simulink model "WithLoad_Simple"  (R2017b)
settings: Solver=ode3  StartTime=0.0  StopTime=10  FixedStep=0.005  RelTol=1e-3  EnableMultiTasking=on
libraries: mblibv1 x61
(part 2 of 3)

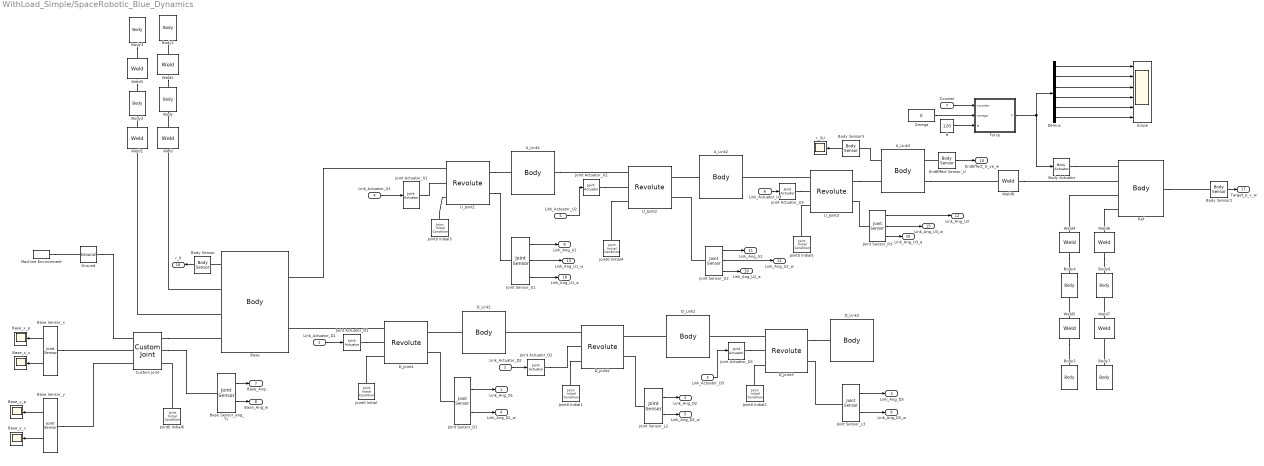
== system WithLoad_Simple/SpaceRobotic_Blue_Dynamics ==
  Link_Actuator_D1 : Inport
  Link_Actuator_D2 : Inport  Port=2
  Link_Actuator_D3 : Inport  Port=3
  Link_Actuator_U1 : Inport  Port=4
  Link_Actuator_U2 : Inport  Port=5
  Link_Actuator_U3 : Inport  Port=6
  Counter : Inport  Port=7
  Base : mblibv1/Bodies/Body  LConnTagsString=CG|CS14|CS15|CS1  RConnTagsString=CS16|CS17  UpdateFromCAD=off  DialogClass=MechanicalBodyBlock  Mass=44.0  MassUnits=kg  InertiaUnits=kg*m^2  Inertia=44.0*eye(3)  Shape=Cylinder  ShapeDims=[1 1]  ShapeUnits=m  ShapeUse=false  Density=1  DensityUnits=kg/m^3  DensityUse=false  GraphicsMode=MACHINE_DEFAULT  BodyColorSelMode=COLORPALETTE  BodyColor=[1 0.69412 0.39216]  AttachedToCS=CG  CG=Left$CG$[0.0 0 0]$CS1$CS1$m$[0 0 0]$Euler X-Y-Z$deg$WORLD$true$none  WorkingFrames=Left$CS14$[0 0 0.3]$CS1$CS1$m$[0 0 0]$Euler X-Y-Z$deg$WORLD$true$none#Left$CS15$[0 0 -0.3]$CS1$CS1$m$[0 0 0]$Euler X-Y-Z$deg$WORLD$true$none#Left$CS1$[0 0 0]$Adjoining$Adjoining$m$[0 0 0]$Euler X-Y-Z$deg$WORLD$true$none#Left$CS5$[-0.3 -0.3 0]$CS1$CS1$m$[0 0 0]$Euler X-Y-Z$deg$WORLD$false$none#Left$CS4$[-0.3 0.3 0]$CS1$CS1$m$[0 0 0]$Euler X-Y-Z$deg$WORLD$false$none#Right$CS2$[0.3 0.3 0]$CS1$CS1$m$[0 0 0]$Euler X-Y-Z$deg$WORLD$false$none#Right$CS16$[0.3 0.3 0]$CS1$CS1$m$[0 0 0]$Euler X-Y-Z$deg$WORLD$true$none#Right$CS3$[0.3 -0.3 0]$CS1$CS1$m$[0 0 0]$Euler X-Y-Z$deg$WORLD$false$none#Right$CS17$[0.3 -0.3 0]$CS1$CS1$m$[0 0 0]$Euler X-Y-Z$deg$WORLD$true$none#Right$CS13$[-0.3 0.3 -0.3]$CS1$CS1$m$[0 0 0]$Euler X-Y-Z$deg$WORLD$false$none#Right$CS12$[-0.3 0.3 0.3]$CS1$CS1$m$[0 0 0]$Euler X-Y-Z$deg$WORLD$false$none#Right$CS11$[0.3 0.3 -0.3]$CS1$CS1$m$[0 0 0]$Euler X-Y-Z$deg$WORLD$false$none#Right$CS10$[0.3 0.3 0.3]$CS1$CS1$m$[0 0 0]$Euler X-Y-Z$deg$WORLD$false$none#Right$CS9$[-0.3 -0.3 -0.3]$CS1$CS1$m$[0 0 0]$Euler X-Y-Z$deg$WORLD$false$none#Right$CS8$[0.3 -0.3 -0.3]$CS1$CS1$m$[0 0 0]$Euler X-Y-Z$deg$WORLD$false$none#Right$CS7$[-0.3 -0.3 0.3]$CS1$CS1$m$[0 0 0]$Euler X-Y-Z$deg$WORLD$false$none#Right$CS6$[0.3 -0.3 0.3]$CS1$CS1$m$[0 0 0]$Euler X-Y-Z$deg$WORLD$false$none  CGPos=[0.0 0 0]  CGRot=[0 0 0]  CS0Pos=[]  CS0Rot=[]  CS1Pos=[0 0 0]  CS1Rot=[0 0 0]  CS2Pos=[0.3 0.3 0]  CS2Rot=[0 0 0]  CS3Pos=[0.3 -0.3 0]  CS3Rot=[0 0 0]  CS4Pos=[-0.3 0.3 0]  CS4Rot=[0 0 0]  CS5Pos=[-0.3 -0.3 0]  CS5Rot=[0 0 0]  CS6Pos=[0.3 -0.3 0.3]  CS6Rot=[0 0 0]  CS7Pos=[-0.3 -0.3 0.3]  CS7Rot=[0 0 0]  CS8Pos=[0.3 -0.3 -0.3]  CS8Rot=[0 0 0]  CS9Pos=[-0.3 -0.3 -0.3]  CS9Rot=[0 0 0]  CS10Pos=[0.3 0.3 0.3]  CS10Rot=[0 0 0]  CS11Pos=[0.3 0.3 -0.3]  CS11Rot=[0 0 0]  CS12Pos=[-0.3 0.3 0.3]  CS12Rot=[0 0 0]  CS13Pos=[-0.3 0.3 -0.3]  CS13Rot=[0 0 0]  CS14Pos=[0 0 0.3]  CS14Rot=[0 0 0]  CS15Pos=[0 0 -0.3]  CS15Rot=[0 0 0]  CS16Pos=[0.3 0.3 0]  CS16Rot=[0 0 0]  CS17Pos=[0.3 -0.3 0]  CS17Rot=[0 0 0]  CS18Pos=[]  CS18Rot=[]  CS19Pos=[]  CS19Rot=[]  CS20Pos=[]  CS20Rot=[]
      settings: SourceProductName=Simscape Multibody  SourceProductBaseCode=MS
  Base Sensor_ang_Tc : mblibv1/Sensors &  Actuators/Joint Sensor  UpdateFromCAD=off  PhysicalDomain=Mechanical  PortType=blob  Muxed=off  Pose=off  Angle=on  AngleUnits=rad  ArcVelocity=on  ArcVelocityUnits=rad/s  ArcAcceleration=off  ArcAccelerationUnits=deg/s^2  CoordPosition=on  CoordPositionUnits=m  Velocity=off  VelocityUnits=m/s  Acceleration=off  AccelerationUnits=m/s^2  Quaternion=on  QuaternionDT=off  QuaternionDDT=off  QuaternionUnits=off  OutputVector=[1]  ActiveIO=on  Width=2  DialogClass=MechanicalSensorBlock  Primitive=R1  Force=off  ForceUnits=N  Torque=off  TorqueUnits=N*m  ReferenceFrame=Absolute (World)  ReactionSensedSide=Base  ReactionReferenceFrame=Absolute (World)  ReactionForce=off  ReactionForceUnits=N  ReactionMoment=off  ReactionMomentUnits=N*m
      settings: SourceProductName=Simscape Multibody  SourceProductBaseCode=MS
  Base Sensor_x : mblibv1/Sensors &  Actuators/Joint Sensor  UpdateFromCAD=off  PhysicalDomain=Mechanical  PortType=blob  Muxed=off  Pose=off  Angle=on  AngleUnits=deg  ArcVelocity=on  ArcVelocityUnits=deg/s  ArcAcceleration=off  ArcAccelerationUnits=deg/s^2  CoordPosition=on  CoordPositionUnits=m  Velocity=on  VelocityUnits=m/s  Acceleration=off  AccelerationUnits=m/s^2  Quaternion=on  QuaternionDT=off  QuaternionDDT=off  QuaternionUnits=off  OutputVector=[1]  ActiveIO=on  Width=2  DialogClass=MechanicalSensorBlock  Primitive=P1  Force=off  ForceUnits=N  Torque=off  TorqueUnits=N*m  ReferenceFrame=Absolute (World)  ReactionSensedSide=Base  ReactionReferenceFrame=Absolute (World)  ReactionForce=off  ReactionForceUnits=N  ReactionMoment=off  ReactionMomentUnits=N*m
      settings: SourceProductName=Simscape Multibody  SourceProductBaseCode=MS
  Base Sensor_y : mblibv1/Sensors &  Actuators/Joint Sensor  UpdateFromCAD=off  PhysicalDomain=Mechanical  PortType=blob  Muxed=off  Pose=off  Angle=on  AngleUnits=deg  ArcVelocity=on  ArcVelocityUnits=deg/s  ArcAcceleration=off  ArcAccelerationUnits=deg/s^2  CoordPosition=on  CoordPositionUnits=m  Velocity=on  VelocityUnits=m/s  Acceleration=off  AccelerationUnits=m/s^2  Quaternion=on  QuaternionDT=off  QuaternionDDT=off  QuaternionUnits=off  OutputVector=[1]  ActiveIO=on  Width=2  DialogClass=MechanicalSensorBlock  Primitive=P2  Force=off  ForceUnits=N  Torque=off  TorqueUnits=N*m  ReferenceFrame=Absolute (World)  ReactionSensedSide=Base  ReactionReferenceFrame=Absolute (World)  ReactionForce=off  ReactionForceUnits=N  ReactionMoment=off  ReactionMomentUnits=N*m
      settings: SourceProductName=Simscape Multibody  SourceProductBaseCode=MS
  Base_x_p : Scope
  Base_x_v : Scope
  Base_y_p : Scope
  Base_y_v : Scope
  Body : mblibv1/Bodies/Body  LConnTagsString=CS1  RConnTagsString=CS2  UpdateFromCAD=off  DialogClass=MechanicalBodyBlock  Mass=1*0.00001  MassUnits=kg  InertiaUnits=kg*m^2  Inertia=eye(3)*0.00001*(1)  Shape=Cylinder  ShapeDims=[1 1]  ShapeUnits=m  ShapeUse=false  Density=1  DensityUnits=kg/m^3  DensityUse=false  GraphicsMode=MACHINE_DEFAULT  BodyColorSelMode=COLORPALETTE  BodyColor=[0 0 1]  AttachedToCS=CG  CG=Left$CG$[0 0 0.1]$CS1$CS1$m$[0 0 0]$Euler X-Y-Z$deg$WORLD$false$none  WorkingFrames=Left$CS1$[0 0 0]$Adjoining$Adjoining$m$[0 0 0]$Euler X-Y-Z$deg$WORLD$true$none#Right$CS2$[0 0 0.2]$CS1$CS1$m$[0 0 0]$Euler X-Y-Z$deg$WORLD$true$none  CGPos=[0 0 0.1]  CGRot=[0 0 0]  CS0Pos=[]  CS0Rot=[]  CS1Pos=[0 0 0]  CS1Rot=[0 0 0]  CS2Pos=[0 0 0.2]  CS2Rot=[0 0 0]  CS3Pos=[]  CS3Rot=[]  CS4Pos=[]  CS4Rot=[]  CS5Pos=[]  CS5Rot=[]  CS6Pos=[]  CS6Rot=[]  CS7Pos=[]  CS7Rot=[]  CS8Pos=[]  CS8Rot=[]  CS9Pos=[]  CS9Rot=[]  CS10Pos=[]  CS10Rot=[]  CS11Pos=[]  CS11Rot=[]  CS12Pos=[]  CS12Rot=[]  CS13Pos=[]  CS13Rot=[]  CS14Pos=[]  CS14Rot=[]  CS15Pos=[]  CS15Rot=[]  CS16Pos=[]  CS16Rot=[]  CS17Pos=[]  CS17Rot=[]  CS18Pos=[]  CS18Rot=[]  CS19Pos=[]  CS19Rot=[]  CS20Pos=[]  CS20Rot=[]
      settings: SourceProductName=Simscape Multibody  SourceProductBaseCode=MS
  Body Actuator : mblibv1/Sensors &  Actuators/Body Actuator  UpdateFromCAD=off  PhysicalDomain=Mechanical  PortType=blob  ActuationStyle=Force  AngleUnits=deg  ArcVelocityUnits=deg/s  ArcAccelerationUnits=deg/s^2  CoordPositionUnits=m  VelocityUnits=m/s  AccelerationUnits=m/s^2  ForceUnits=N  TorqueUnits=N*m  ActiveIO=on  Width=6  DialogClass=MechanicalActuatorBlock  ReferenceFrame=Local (Body CS)  Angle=off  CoordPosition=on  Force=on  Torque=on
      settings: SourceProductName=Simscape Multibody  SourceProductBaseCode=MS
  Body Sensor : mblibv1/Sensors &  Actuators/Body Sensor  UpdateFromCAD=off  PhysicalDomain=Mechanical  PortType=blob  Muxed=on  Pose=off  Angle=on  AngleUnits=deg  ArcVelocity=on  ArcVelocityUnits=rad/s  ArcAcceleration=on  ArcAccelerationUnits=deg/s^2  CoordPosition=on  CoordPositionUnits=m  Velocity=on  VelocityUnits=m/s  Acceleration=off  AccelerationUnits=m/s^2  Quaternion=on  QuaternionDT=off  QuaternionDDT=off  QuaternionUnits=off  OutputVector=[1]  ActiveIO=on  Width=12  DialogClass=MechanicalSensorBlock  ReferenceFrame=Absolute (World)
      settings: SourceProductName=Simscape Multibody  SourceProductBaseCode=MS
  Body Sensor2 : mblibv1/Sensors &  Actuators/Body Sensor  UpdateFromCAD=off  PhysicalDomain=Mechanical  PortType=blob  Muxed=on  Pose=off  Angle=on  AngleUnits=deg  ArcVelocity=on  ArcVelocityUnits=rad/s  ArcAcceleration=off  ArcAccelerationUnits=deg/s^2  CoordPosition=on  CoordPositionUnits=m  Velocity=on  VelocityUnits=m/s  Acceleration=off  AccelerationUnits=m/s^2  Quaternion=on  QuaternionDT=off  QuaternionDDT=off  QuaternionUnits=off  OutputVector=[1]  ActiveIO=on  Width=9  DialogClass=MechanicalSensorBlock  ReferenceFrame=Absolute (World)
      settings: SourceProductName=Simscape Multibody  SourceProductBaseCode=MS
  Body Sensor5 : mblibv1/Sensors &  Actuators/Body Sensor  UpdateFromCAD=off  PhysicalDomain=Mechanical  PortType=blob  Muxed=on  Pose=off  Angle=on  AngleUnits=deg  ArcVelocity=off  ArcVelocityUnits=deg/s  ArcAcceleration=off  ArcAccelerationUnits=deg/s^2  CoordPosition=on  CoordPositionUnits=m  Velocity=off  VelocityUnits=m/s  Acceleration=off  AccelerationUnits=m/s^2  Quaternion=on  QuaternionDT=off  QuaternionDDT=off  QuaternionUnits=off  OutputVector=[1]  ActiveIO=on  Width=3  DialogClass=MechanicalSensorBlock  ReferenceFrame=Absolute (World)
      settings: SourceProductName=Simscape Multibody  SourceProductBaseCode=MS
  Body1 : mblibv1/Bodies/Body  LConnTagsString=CS1  UpdateFromCAD=off  DialogClass=MechanicalBodyBlock  Mass=1*0.00001  MassUnits=kg  InertiaUnits=kg*m^2  Inertia=eye(3)*0.00001  Shape=Cylinder  ShapeDims=[1 1]  ShapeUnits=m  ShapeUse=false  Density=1  DensityUnits=kg/m^3  DensityUse=false  GraphicsMode=MACHINE_DEFAULT  BodyColorSelMode=COLORPALETTE  BodyColor=[0 0 1]  AttachedToCS=CG  CG=Left$CG$[0 0 0.45]$CS1$CS1$m$[0 0 0]$Euler X-Y-Z$deg$WORLD$false$none  WorkingFrames=Left$CS1$[0 0 0]$Adjoining$Adjoining$m$[0 0 0]$Euler X-Y-Z$deg$WORLD$true$none#Right$CS2$[0.2 0.01 0]$CS1$CS1$m$[0 0 0]$Euler X-Y-Z$deg$WORLD$false$none#Right$CS3$[0.2 -0.01 0]$CS1$CS1$m$[0 0 0]$Euler X-Y-Z$deg$WORLD$false$none#Right$CS4$[-0.2 0.01 0]$CS1$CS1$m$[0 0 0]$Euler X-Y-Z$deg$WORLD$false$none#Right$CS5$[-0.2 -0.01 0]$CS1$CS1$m$[0 0 0]$Euler X-Y-Z$deg$WORLD$false$none#Right$CS6$[-0.2 -0.01 0.9]$CS1$CS1$m$[0 0 0]$Euler X-Y-Z$deg$WORLD$false$none#Right$CS7$[-0.2 0.01 0.9]$CS1$CS1$m$[0 0 0]$Euler X-Y-Z$deg$WORLD$false$none#Right$CS8$[0.2 0.01 0.9]$CS1$CS1$m$[0 0 0]$Euler X-Y-Z$deg$WORLD$false$none#Right$CS9$[0.2 -0.01 0.9]$CS1$CS1$m$[0 0 0]$Euler X-Y-Z$deg$WORLD$false$none  CGPos=[0 0 0.45]  CGRot=[0 0 0]  CS0Pos=[]  CS0Rot=[]  CS1Pos=[0 0 0]  CS1Rot=[0 0 0]  CS2Pos=[0.2 0.01 0]  CS2Rot=[0 0 0]  CS3Pos=[0.2 -0.01 0]  CS3Rot=[0 0 0]  CS4Pos=[-0.2 0.01 0]  CS4Rot=[0 0 0]  CS5Pos=[-0.2 -0.01 0]  CS5Rot=[0 0 0]  CS6Pos=[-0.2 -0.01 0.9]  CS6Rot=[0 0 0]  CS7Pos=[-0.2 0.01 0.9]  CS7Rot=[0 0 0]  CS8Pos=[0.2 0.01 0.9]  CS8Rot=[0 0 0]  CS9Pos=[0.2 -0.01 0.9]  CS9Rot=[0 0 0]  CS10Pos=[]  CS10Rot=[]  CS11Pos=[]  CS11Rot=[]  CS12Pos=[]  CS12Rot=[]  CS13Pos=[]  CS13Rot=[]  CS14Pos=[]  CS14Rot=[]  CS15Pos=[]  CS15Rot=[]  CS16Pos=[]  CS16Rot=[]  CS17Pos=[]  CS17Rot=[]  CS18Pos=[]  CS18Rot=[]  CS19Pos=[]  CS19Rot=[]  CS20Pos=[]  CS20Rot=[]
      settings: SourceProductName=Simscape Multibody  SourceProductBaseCode=MS
  Body2 : mblibv1/Bodies/Body  LConnTagsString=CS1  RConnTagsString=CS2  UpdateFromCAD=off  DialogClass=MechanicalBodyBlock  Mass=1*0.00001  MassUnits=kg  InertiaUnits=kg*m^2  Inertia=eye(3)*0.00001  Shape=Cylinder  ShapeDims=[1 1]  ShapeUnits=m  ShapeUse=false  Density=1  DensityUnits=kg/m^3  DensityUse=false  GraphicsMode=MACHINE_DEFAULT  BodyColorSelMode=COLORPALETTE  BodyColor=[0 0 1]  AttachedToCS=CG  CG=Left$CG$[0 0 -0.1]$CS1$CS1$m$[0 0 0]$Euler X-Y-Z$deg$WORLD$false$none  WorkingFrames=Left$CS1$[0 0 0]$Adjoining$Adjoining$m$[0 0 0]$Euler X-Y-Z$deg$WORLD$true$none#Right$CS2$[0 0 -0.2]$CS1$CS1$m$[0 0 0]$Euler X-Y-Z$deg$WORLD$true$none  CGPos=[0 0 -0.1]  CGRot=[0 0 0]  CS0Pos=[]  CS0Rot=[]  CS1Pos=[0 0 0]  CS1Rot=[0 0 0]  CS2Pos=[0 0 -0.2]  CS2Rot=[0 0 0]  CS3Pos=[]  CS3Rot=[]  CS4Pos=[]  CS4Rot=[]  CS5Pos=[]  CS5Rot=[]  CS6Pos=[]  CS6Rot=[]  CS7Pos=[]  CS7Rot=[]  CS8Pos=[]  CS8Rot=[]  CS9Pos=[]  CS9Rot=[]  CS10Pos=[]  CS10Rot=[]  CS11Pos=[]  CS11Rot=[]  CS12Pos=[]  CS12Rot=[]  CS13Pos=[]  CS13Rot=[]  CS14Pos=[]  CS14Rot=[]  CS15Pos=[]  CS15Rot=[]  CS16Pos=[]  CS16Rot=[]  CS17Pos=[]  CS17Rot=[]  CS18Pos=[]  CS18Rot=[]  CS19Pos=[]  CS19Rot=[]  CS20Pos=[]  CS20Rot=[]
      settings: SourceProductName=Simscape Multibody  SourceProductBaseCode=MS
  Body3 : mblibv1/Bodies/Body  LConnTagsString=CS1  UpdateFromCAD=off  DialogClass=MechanicalBodyBlock  Mass=1*0.00001  MassUnits=kg  InertiaUnits=kg*m^2  Inertia=eye(3)*0.00001  Shape=Cylinder  ShapeDims=[1 1]  ShapeUnits=m  ShapeUse=false  Density=1  DensityUnits=kg/m^3  DensityUse=false  GraphicsMode=MACHINE_DEFAULT  BodyColorSelMode=COLORPALETTE  BodyColor=[0 0 1]  AttachedToCS=CG  CG=Left$CG$[0 0 0.45]$CS1$CS1$m$[0 0 0]$Euler X-Y-Z$deg$WORLD$false$none  WorkingFrames=Left$CS1$[0 0 0]$Adjoining$Adjoining$m$[0 0 0]$Euler X-Y-Z$deg$WORLD$true$none#Right$CS2$[0.2 0.01 0]$CS1$CS1$m$[0 0 0]$Euler X-Y-Z$deg$WORLD$false$none#Right$CS3$[0.2 -0.01 0]$CS1$CS1$m$[0 0 0]$Euler X-Y-Z$deg$WORLD$false$none#Right$CS4$[-0.2 0.01 0]$CS1$CS1$m$[0 0 0]$Euler X-Y-Z$deg$WORLD$false$none#Right$CS5$[-0.2 -0.01 0]$CS1$CS1$m$[0 0 0]$Euler X-Y-Z$deg$WORLD$false$none#Right$CS6$[-0.2 -0.01 -0.9]$CS1$CS1$m$[0 0 0]$Euler X-Y-Z$deg$WORLD$false$none#Right$CS7$[-0.2 0.01 -0.9]$CS1$CS1$m$[0 0 0]$Euler X-Y-Z$deg$WORLD$false$none#Right$CS8$[0.2 0.01 -0.9]$CS1$CS1$m$[0 0 0]$Euler X-Y-Z$deg$WORLD$false$none#Right$CS9$[0.2 -0.01 -0.9]$CS1$CS1$m$[0 0 0]$Euler X-Y-Z$deg$WORLD$false$none  CGPos=[0 0 0.45]  CGRot=[0 0 0]  CS0Pos=[]  CS0Rot=[]  CS1Pos=[0 0 0]  CS1Rot=[0 0 0]  CS2Pos=[0.2 0.01 0]  CS2Rot=[0 0 0]  CS3Pos=[0.2 -0.01 0]  CS3Rot=[0 0 0]  CS4Pos=[-0.2 0.01 0]  CS4Rot=[0 0 0]  CS5Pos=[-0.2 -0.01 0]  CS5Rot=[0 0 0]  CS6Pos=[-0.2 -0.01 -0.9]  CS6Rot=[0 0 0]  CS7Pos=[-0.2 0.01 -0.9]  CS7Rot=[0 0 0]  CS8Pos=[0.2 0.01 -0.9]  CS8Rot=[0 0 0]  CS9Pos=[0.2 -0.01 -0.9]  CS9Rot=[0 0 0]  CS10Pos=[]  CS10Rot=[]  CS11Pos=[]  CS11Rot=[]  CS12Pos=[]  CS12Rot=[]  CS13Pos=[]  CS13Rot=[]  CS14Pos=[]  CS14Rot=[]  CS15Pos=[]  CS15Rot=[]  CS16Pos=[]  CS16Rot=[]  CS17Pos=[]  CS17Rot=[]  CS18Pos=[]  CS18Rot=[]  CS19Pos=[]  CS19Rot=[]  CS20Pos=[]  CS20Rot=[]
      settings: SourceProductName=Simscape Multibody  SourceProductBaseCode=MS
  Body4 : mblibv1/Bodies/Body  LConnTagsString=CS1  RConnTagsString=CS2  UpdateFromCAD=off  DialogClass=MechanicalBodyBlock  Mass=1*0.00001  MassUnits=kg  InertiaUnits=kg*m^2  Inertia=eye(3)*0.00001  Shape=Cylinder  ShapeDims=[1 1]  ShapeUnits=m  ShapeUse=false  Density=1  DensityUnits=kg/m^3  DensityUse=false  GraphicsMode=MACHINE_DEFAULT  BodyColorSelMode=COLORPALETTE  BodyColor=[0 0 1]  AttachedToCS=CG  CG=Left$CG$[0 0 0.1]$CS1$CS1$m$[0 0 0]$Euler X-Y-Z$deg$WORLD$false$none  WorkingFrames=Left$CS1$[0 0 0]$Adjoining$Adjoining$m$[0 0 0]$Euler X-Y-Z$deg$WORLD$true$none#Right$CS2$[0 0 0.2]$CS1$CS1$m$[0 0 0]$Euler X-Y-Z$deg$WORLD$true$none  CGPos=[0 0 0.1]  CGRot=[0 0 0]  CS0Pos=[]  CS0Rot=[]  CS1Pos=[0 0 0]  CS1Rot=[0 0 0]  CS2Pos=[0 0 0.2]  CS2Rot=[0 0 0]  CS3Pos=[]  CS3Rot=[]  CS4Pos=[]  CS4Rot=[]  CS5Pos=[]  CS5Rot=[]  CS6Pos=[]  CS6Rot=[]  CS7Pos=[]  CS7Rot=[]  CS8Pos=[]  CS8Rot=[]  CS9Pos=[]  CS9Rot=[]  CS10Pos=[]  CS10Rot=[]  CS11Pos=[]  CS11Rot=[]  CS12Pos=[]  CS12Rot=[]  CS13Pos=[]  CS13Rot=[]  CS14Pos=[]  CS14Rot=[]  CS15Pos=[]  CS15Rot=[]  CS16Pos=[]  CS16Rot=[]  CS17Pos=[]  CS17Rot=[]  CS18Pos=[]  CS18Rot=[]  CS19Pos=[]  CS19Rot=[]  CS20Pos=[]  CS20Rot=[]
      settings: SourceProductName=Simscape Multibody  SourceProductBaseCode=MS
  Body5 : mblibv1/Bodies/Body  LConnTagsString=CS1  UpdateFromCAD=off  DialogClass=MechanicalBodyBlock  Mass=1*0.00001  MassUnits=kg  InertiaUnits=kg*m^2  Inertia=eye(3)*0.00001  Shape=Cylinder  ShapeDims=[1 1]  ShapeUnits=m  ShapeUse=false  Density=1  DensityUnits=kg/m^3  DensityUse=false  GraphicsMode=MACHINE_DEFAULT  BodyColorSelMode=COLORPALETTE  BodyColor=[0 0 1]  AttachedToCS=CG  CG=Left$CG$[0 0 0.45]$CS1$CS1$m$[0 0 0]$Euler X-Y-Z$deg$WORLD$false$none  WorkingFrames=Left$CS1$[0 0 0]$Adjoining$Adjoining$m$[0 0 0]$Euler X-Y-Z$deg$WORLD$true$none#Right$CS2$[0.2 0.01 0]$CS1$CS1$m$[0 0 0]$Euler X-Y-Z$deg$WORLD$false$none#Right$CS3$[0.2 -0.01 0]$CS1$CS1$m$[0 0 0]$Euler X-Y-Z$deg$WORLD$false$none#Right$CS4$[-0.2 0.01 0]$CS1$CS1$m$[0 0 0]$Euler X-Y-Z$deg$WORLD$false$none#Right$CS5$[-0.2 -0.01 0]$CS1$CS1$m$[0 0 0]$Euler X-Y-Z$deg$WORLD$false$none#Right$CS6$[-0.2 -0.01 1]$CS1$CS1$m$[0 0 0]$Euler X-Y-Z$deg$WORLD$false$none#Right$CS7$[-0.2 0.01 1]$CS1$CS1$m$[0 0 0]$Euler X-Y-Z$deg$WORLD$false$none#Right$CS8$[0.2 0.01 1]$CS1$CS1$m$[0 0 0]$Euler X-Y-Z$deg$WORLD$false$none#Right$CS9$[0.2 -0.01 1]$CS1$CS1$m$[0 0 0]$Euler X-Y-Z$deg$WORLD$false$none  CGPos=[0 0 0.45]  CGRot=[0 0 0]  CS0Pos=[]  CS0Rot=[]  CS1Pos=[0 0 0]  CS1Rot=[0 0 0]  CS2Pos=[0.2 0.01 0]  CS2Rot=[0 0 0]  CS3Pos=[0.2 -0.01 0]  CS3Rot=[0 0 0]  CS4Pos=[-0.2 0.01 0]  CS4Rot=[0 0 0]  CS5Pos=[-0.2 -0.01 0]  CS5Rot=[0 0 0]  CS6Pos=[-0.2 -0.01 1]  CS6Rot=[0 0 0]  CS7Pos=[-0.2 0.01 1]  CS7Rot=[0 0 0]  CS8Pos=[0.2 0.01 1]  CS8Rot=[0 0 0]  CS9Pos=[0.2 -0.01 1]  CS9Rot=[0 0 0]  CS10Pos=[]  CS10Rot=[]  CS11Pos=[]  CS11Rot=[]  CS12Pos=[]  CS12Rot=[]  CS13Pos=[]  CS13Rot=[]  CS14Pos=[]  CS14Rot=[]  CS15Pos=[]  CS15Rot=[]  CS16Pos=[]  CS16Rot=[]  CS17Pos=[]  CS17Rot=[]  CS18Pos=[]  CS18Rot=[]  CS19Pos=[]  CS19Rot=[]  CS20Pos=[]  CS20Rot=[]
      settings: SourceProductName=Simscape Multibody  SourceProductBaseCode=MS
  Body6 : mblibv1/Bodies/Body  LConnTagsString=CS1  RConnTagsString=CS2  UpdateFromCAD=off  DialogClass=MechanicalBodyBlock  Mass=1*0.00001  MassUnits=kg  InertiaUnits=kg*m^2  Inertia=eye(3)*0.00001  Shape=Cylinder  ShapeDims=[1 1]  ShapeUnits=m  ShapeUse=false  Density=1  DensityUnits=kg/m^3  DensityUse=false  GraphicsMode=MACHINE_DEFAULT  BodyColorSelMode=COLORPALETTE  BodyColor=[0 0 1]  AttachedToCS=CG  CG=Left$CG$[0 0 -0.1]$CS1$CS1$m$[0 0 0]$Euler X-Y-Z$deg$WORLD$false$none  WorkingFrames=Left$CS1$[0 0 0]$Adjoining$Adjoining$m$[0 0 0]$Euler X-Y-Z$deg$WORLD$true$none#Right$CS2$[0 0 -0.2]$CS1$CS1$m$[0 0 0]$Euler X-Y-Z$deg$WORLD$true$none  CGPos=[0 0 -0.1]  CGRot=[0 0 0]  CS0Pos=[]  CS0Rot=[]  CS1Pos=[0 0 0]  CS1Rot=[0 0 0]  CS2Pos=[0 0 -0.2]  CS2Rot=[0 0 0]  CS3Pos=[]  CS3Rot=[]  CS4Pos=[]  CS4Rot=[]  CS5Pos=[]  CS5Rot=[]  CS6Pos=[]  CS6Rot=[]  CS7Pos=[]  CS7Rot=[]  CS8Pos=[]  CS8Rot=[]  CS9Pos=[]  CS9Rot=[]  CS10Pos=[]  CS10Rot=[]  CS11Pos=[]  CS11Rot=[]  CS12Pos=[]  CS12Rot=[]  CS13Pos=[]  CS13Rot=[]  CS14Pos=[]  CS14Rot=[]  CS15Pos=[]  CS15Rot=[]  CS16Pos=[]  CS16Rot=[]  CS17Pos=[]  CS17Rot=[]  CS18Pos=[]  CS18Rot=[]  CS19Pos=[]  CS19Rot=[]  CS20Pos=[]  CS20Rot=[]
      settings: SourceProductName=Simscape Multibody  SourceProductBaseCode=MS
  Body7 : mblibv1/Bodies/Body  LConnTagsString=CS1  UpdateFromCAD=off  DialogClass=MechanicalBodyBlock  Mass=1*0.00001  MassUnits=kg  InertiaUnits=kg*m^2  Inertia=eye(3)*0.00001  Shape=Cylinder  ShapeDims=[1 1]  ShapeUnits=m  ShapeUse=false  Density=1  DensityUnits=kg/m^3  DensityUse=false  GraphicsMode=MACHINE_DEFAULT  BodyColorSelMode=COLORPALETTE  BodyColor=[0 0 1]  AttachedToCS=CG  CG=Left$CG$[0 0 0.45]$CS1$CS1$m$[0 0 0]$Euler X-Y-Z$deg$WORLD$false$none  WorkingFrames=Left$CS1$[0 0 0]$Adjoining$Adjoining$m$[0 0 0]$Euler X-Y-Z$deg$WORLD$true$none#Right$CS2$[0.2 0.01 0]$CS1$CS1$m$[0 0 0]$Euler X-Y-Z$deg$WORLD$false$none#Right$CS3$[0.2 -0.01 0]$CS1$CS1$m$[0 0 0]$Euler X-Y-Z$deg$WORLD$false$none#Right$CS4$[-0.2 0.01 0]$CS1$CS1$m$[0 0 0]$Euler X-Y-Z$deg$WORLD$false$none#Right$CS5$[-0.2 -0.01 0]$CS1$CS1$m$[0 0 0]$Euler X-Y-Z$deg$WORLD$false$none#Right$CS6$[-0.2 -0.01 -1]$CS1$CS1$m$[0 0 0]$Euler X-Y-Z$deg$WORLD$false$none#Right$CS7$[-0.2 0.01 -1]$CS1$CS1$m$[0 0 0]$Euler X-Y-Z$deg$WORLD$false$none#Right$CS8$[0.2 0.01 -1]$CS1$CS1$m$[0 0 0]$Euler X-Y-Z$deg$WORLD$false$none#Right$CS9$[0.2 -0.01 -1]$CS1$CS1$m$[0 0 0]$Euler X-Y-Z$deg$WORLD$false$none  CGPos=[0 0 0.45]  CGRot=[0 0 0]  CS0Pos=[]  CS0Rot=[]  CS1Pos=[0 0 0]  CS1Rot=[0 0 0]  CS2Pos=[0.2 0.01 0]  CS2Rot=[0 0 0]  CS3Pos=[0.2 -0.01 0]  CS3Rot=[0 0 0]  CS4Pos=[-0.2 0.01 0]  CS4Rot=[0 0 0]  CS5Pos=[-0.2 -0.01 0]  CS5Rot=[0 0 0]  CS6Pos=[-0.2 -0.01 -1]  CS6Rot=[0 0 0]  CS7Pos=[-0.2 0.01 -1]  CS7Rot=[0 0 0]  CS8Pos=[0.2 0.01 -1]  CS8Rot=[0 0 0]  CS9Pos=[0.2 -0.01 -1]  CS9Rot=[0 0 0]  CS10Pos=[]  CS10Rot=[]  CS11Pos=[]  CS11Rot=[]  CS12Pos=[]  CS12Rot=[]  CS13Pos=[]  CS13Rot=[]  CS14Pos=[]  CS14Rot=[]  CS15Pos=[]  CS15Rot=[]  CS16Pos=[]  CS16Rot=[]  CS17Pos=[]  CS17Rot=[]  CS18Pos=[]  CS18Rot=[]  CS19Pos=[]  CS19Rot=[]  CS20Pos=[]  CS20Rot=[]
      settings: SourceProductName=Simscape Multibody  SourceProductBaseCode=MS
  Custom Joint : mblibv1/Joints/Custom Joint  LConnTagsString=__newl0|SA1|SA2  RConnTagsString=__newr0|SA1|SA2  UpdateFromCAD=off  NumSAPorts=4  CutJoint=off  MarkAsCut=off  Primitives=prismatic  PrimitiveProps=R1$World$[0 0 1]$revolute#P1$World$[1 0 0]$Prismatic#P2$World$[0 1 0]$Prismatic  DialogClass=JointBlock  R1Axis=[0 0 1]  R2Axis=[]  R3Axis=[]  P1Axis=[1 0 0]  P2Axis=[0 1 0]  P3Axis=[]  SAxis=[]
      settings: SourceProductName=Simscape Multibody  SourceProductBaseCode=MS
  D_Joint1 : mblibv1/Joints/Revolute  LConnTagsString=__newl0|SA1|SA2  RConnTagsString=__newr0|SA1  UpdateFromCAD=off  NumSAPorts=3  CutJoint=off  MarkAsCut=off  Primitives=prismatic  PrimitiveProps=R1$World$[0 0 1]$revolute  DialogClass=JointBlock  R1Axis=[0 0 1]
      settings: SourceProductName=Simscape Multibody  SourceProductBaseCode=MS
  D_Joint2 : mblibv1/Joints/Revolute  LConnTagsString=__newl0|SA1|SA2  RConnTagsString=__newr0|SA1  UpdateFromCAD=off  NumSAPorts=3  CutJoint=off  MarkAsCut=off  Primitives=prismatic  PrimitiveProps=R1$World$[0 0 1]$revolute  DialogClass=JointBlock  R1Axis=[0 0 1]
      settings: SourceProductName=Simscape Multibody  SourceProductBaseCode=MS
  D_Joint3 : mblibv1/Joints/Revolute  LConnTagsString=__newl0|SA1|SA2  RConnTagsString=__newr0|SA1  UpdateFromCAD=off  NumSAPorts=3  CutJoint=off  MarkAsCut=off  Primitives=prismatic  PrimitiveProps=R1$World$[0 0 1]$revolute  DialogClass=JointBlock  R1Axis=[0 0 1]
      settings: SourceProductName=Simscape Multibody  SourceProductBaseCode=MS
  D_Link1 : mblibv1/Bodies/Body  LConnTagsString=CS2  RConnTagsString=CS1  UpdateFromCAD=off  DialogClass=MechanicalBodyBlock  Mass=2.49  MassUnits=kg  InertiaUnits=kg*m^2  Inertia=[0.208 0 0; 0 0.208 0;0 0 0.208]  Shape=Cylinder  ShapeDims=[1 1]  ShapeUnits=m  ShapeUse=false  Density=1  DensityUnits=kg/m^3  DensityUse=false  GraphicsMode=MACHINE_DEFAULT  BodyColorSelMode=COLORPALETTE  BodyColor=[0 0.8 0.8]  AttachedToCS=CG  CG=Right$CG$[0.2 0.0 0]$CS1$CS1$m$[0 0 0]$Euler X-Y-Z$deg$WORLD$false$none  WorkingFrames=Right$CS1$[0 0 0]$Adjoining$Adjoining$m$[0 0 0]$Euler X-Y-Z$deg$WORLD$true$none#Left$CS2$[0.4 0.0 0]$CS1$CS1$m$[0 0 0]$Euler X-Y-Z$deg$WORLD$true$none#Left$CS3$[0.4 0.02 0.02]$CS1$CS1$m$[0 0 0]$Euler X-Y-Z$deg$WORLD$false$none#Left$CS7$[0.0 0.02 0.02]$CS1$CS1$m$[0 0 0]$Euler X-Y-Z$deg$WORLD$false$none#Left$CS6$[0.4 -0.02 -0.02]$CS1$CS1$m$[0 0 0]$Euler X-Y-Z$deg$WORLD$false$none#Left$CS8$[0.0 -0.02 -0.02]$CS1$CS1$m$[0 0 0]$Euler X-Y-Z$deg$WORLD$false$none#Left$CS5$[0.4 0.02 -0.02]$CS1$CS1$m$[0 0 0]$Euler X-Y-Z$deg$WORLD$false$none#Left$CS9$[0.0 0.02 -0.02]$CS1$CS1$m$[0 0 0]$Euler X-Y-Z$deg$WORLD$false$none#Left$CS4$[0.4 -0.02 0.02]$CS1$CS1$m$[0 0 0]$Euler X-Y-Z$deg$WORLD$false$none#Left$CS10$[0.0 -0.02 0.02]$CS1$CS1$m$[0 0 0]$Euler X-Y-Z$deg$WORLD$false$none  CGPos=[0.2 0.0 0]  CGRot=[0 0 0]  CS0Pos=[]  CS0Rot=[]  CS1Pos=[0 0 0]  CS1Rot=[0 0 0]  CS2Pos=[0.4 0.0 0]  CS2Rot=[0 0 0]  CS3Pos=[0.4 0.02 0.02]  CS3Rot=[0 0 0]  CS4Pos=[0.4 -0.02 0.02]  CS4Rot=[0 0 0]  CS5Pos=[0.4 0.02 -0.02]  CS5Rot=[0 0 0]  CS6Pos=[0.4 -0.02 -0.02]  CS6Rot=[0 0 0]  CS7Pos=[0.0 0.02 0.02]  CS7Rot=[0 0 0]  CS8Pos=[0.0 -0.02 -0.02]  CS8Rot=[0 0 0]  CS9Pos=[0.0 0.02 -0.02]  CS9Rot=[0 0 0]  CS10Pos=[0.0 -0.02 0.02]  CS10Rot=[0 0 0]  CS11Pos=[]  CS11Rot=[]  CS12Pos=[]  CS12Rot=[]  CS13Pos=[]  CS13Rot=[]  CS14Pos=[]  CS14Rot=[]  CS15Pos=[]  CS15Rot=[]  CS16Pos=[]  CS16Rot=[]  CS17Pos=[]  CS17Rot=[]  CS18Pos=[]  CS18Rot=[]  CS19Pos=[]  CS19Rot=[]  CS20Pos=[]  CS20Rot=[]
      settings: SourceProductName=Simscape Multibody  SourceProductBaseCode=MS
  D_Link2 : mblibv1/Bodies/Body  LConnTagsString=CS2  RConnTagsString=CS1  UpdateFromCAD=off  DialogClass=MechanicalBodyBlock  Mass=2.49  MassUnits=kg  InertiaUnits=kg*m^2  Inertia=[0.208 0 0; 0 0.208 0;0 0 0.208]  Shape=Cylinder  ShapeDims=[1 1]  ShapeUnits=m  ShapeUse=false  Density=1  DensityUnits=kg/m^3  DensityUse=false  GraphicsMode=MACHINE_DEFAULT  BodyColorSelMode=COLORPALETTE  BodyColor=[0.84706 0.16078 0]  AttachedToCS=CG  CG=Right$CG$[0.2 0.0 0]$CS1$CS1$m$[0 0 0]$Euler X-Y-Z$deg$WORLD$false$none  WorkingFrames=Right$CS1$[0 0 0]$Adjoining$Adjoining$m$[0 0 0]$Euler X-Y-Z$deg$WORLD$true$none#Left$CS2$[0.4 0.0 0]$CS1$CS1$m$[0 0 0]$Euler X-Y-Z$deg$WORLD$true$none#Left$CS3$[0.4 0.02 0.02]$CS1$CS1$m$[0 0 0]$Euler X-Y-Z$deg$WORLD$false$none#Left$CS7$[0.0 0.02 0.02]$CS1$CS1$m$[0 0 0]$Euler X-Y-Z$deg$WORLD$false$none#Left$CS6$[0.4 -0.02 -0.02]$CS1$CS1$m$[0 0 0]$Euler X-Y-Z$deg$WORLD$false$none#Left$CS8$[0.0 -0.02 -0.02]$CS1$CS1$m$[0 0 0]$Euler X-Y-Z$deg$WORLD$false$none#Left$CS5$[0.4 0.02 -0.02]$CS1$CS1$m$[0 0 0]$Euler X-Y-Z$deg$WORLD$false$none#Left$CS9$[0.0 0.02 -0.02]$CS1$CS1$m$[0 0 0]$Euler X-Y-Z$deg$WORLD$false$none#Left$CS4$[0.4 -0.02 0.02]$CS1$CS1$m$[0 0 0]$Euler X-Y-Z$deg$WORLD$false$none#Left$CS10$[0.0 -0.02 0.02]$CS1$CS1$m$[0 0 0]$Euler X-Y-Z$deg$WORLD$false$none  CGPos=[0.2 0.0 0]  CGRot=[0 0 0]  CS0Pos=[]  CS0Rot=[]  CS1Pos=[0 0 0]  CS1Rot=[0 0 0]  CS2Pos=[0.4 0.0 0]  CS2Rot=[0 0 0]  CS3Pos=[0.4 0.02 0.02]  CS3Rot=[0 0 0]  CS4Pos=[0.4 -0.02 0.02]  CS4Rot=[0 0 0]  CS5Pos=[0.4 0.02 -0.02]  CS5Rot=[0 0 0]  CS6Pos=[0.4 -0.02 -0.02]  CS6Rot=[0 0 0]  CS7Pos=[0.0 0.02 0.02]  CS7Rot=[0 0 0]  CS8Pos=[0.0 -0.02 -0.02]  CS8Rot=[0 0 0]  CS9Pos=[0.0 0.02 -0.02]  CS9Rot=[0 0 0]  CS10Pos=[0.0 -0.02 0.02]  CS10Rot=[0 0 0]  CS11Pos=[]  CS11Rot=[]  CS12Pos=[]  CS12Rot=[]  CS13Pos=[]  CS13Rot=[]  CS14Pos=[]  CS14Rot=[]  CS15Pos=[]  CS15Rot=[]  CS16Pos=[]  CS16Rot=[]  CS17Pos=[]  CS17Rot=[]  CS18Pos=[]  CS18Rot=[]  CS19Pos=[]  CS19Rot=[]  CS20Pos=[]  CS20Rot=[]
      settings: SourceProductName=Simscape Multibody  SourceProductBaseCode=MS
  D_Link3 : mblibv1/Bodies/Body  RConnTagsString=CS1  UpdateFromCAD=off  DialogClass=MechanicalBodyBlock  Mass=2.49  MassUnits=kg  InertiaUnits=kg*m^2  Inertia=[0.208 0 0; 0 0.208 0;0 0 0.208]  Shape=Cylinder  ShapeDims=[1 1]  ShapeUnits=m  ShapeUse=false  Density=1  DensityUnits=kg/m^3  DensityUse=false  GraphicsMode=MACHINE_DEFAULT  BodyColorSelMode=COLORPALETTE  BodyColor=[1 1 0]  AttachedToCS=CG  CG=Right$CG$[0.2 0 0]$CS1$CS1$m$[0 0 0]$Euler X-Y-Z$deg$WORLD$false$none  WorkingFrames=Right$CS1$[0 0 0]$Adjoining$Adjoining$m$[0 0 0]$Euler X-Y-Z$deg$WORLD$true$none#Left$CS2$[0.4 0.0 0.0]$CS1$CS1$m$[0 0 0]$Euler X-Y-Z$deg$WORLD$false$none#Left$CS10$[0.4 0.02 0.02]$CS1$CS1$m$[0 0 0]$Euler X-Y-Z$deg$WORLD$false$none#Left$CS3$[0.4 0.02 -0.02]$CS1$CS1$m$[0 0 0]$Euler X-Y-Z$deg$WORLD$false$none#Left$CS4$[0.4 -0.02 -0.02]$CS1$CS1$m$[0 0 0]$Euler X-Y-Z$deg$WORLD$false$none#Left$CS5$[0.4 -0.02 0.02]$CS1$CS1$m$[0 0 0]$Euler X-Y-Z$deg$WORLD$false$none#Left$CS6$[0.0 0.02 0.02]$CS1$CS1$m$[0 0 0]$Euler X-Y-Z$deg$WORLD$false$none#Left$CS9$[0.0 0.02 -0.02]$CS1$CS1$m$[0 0 0]$Euler X-Y-Z$deg$WORLD$false$none#Left$CS8$[0.0 -0.02 0.02]$CS1$CS1$m$[0 0 0]$Euler X-Y-Z$deg$WORLD$false$none#Left$CS7$[0.0 -0.02 -0.02]$CS1$CS1$m$[0 0 0]$Euler X-Y-Z$deg$WORLD$false$none  CGPos=[0.2 0 0]  CGRot=[0 0 0]  CS0Pos=[]  CS0Rot=[]  CS1Pos=[0 0 0]  CS1Rot=[0 0 0]  CS2Pos=[0.4 0.0 0.0]  CS2Rot=[0 0 0]  CS3Pos=[0.4 0.02 -0.02]  CS3Rot=[0 0 0]  CS4Pos=[0.4 -0.02 -0.02]  CS4Rot=[0 0 0]  CS5Pos=[0.4 -0.02 0.02]  CS5Rot=[0 0 0]  CS6Pos=[0.0 0.02 0.02]  CS6Rot=[0 0 0]  CS7Pos=[0.0 -0.02 -0.02]  CS7Rot=[0 0 0]  CS8Pos=[0.0 -0.02 0.02]  CS8Rot=[0 0 0]  CS9Pos=[0.0 0.02 -0.02]  CS9Rot=[0 0 0]  CS10Pos=[0.4 0.02 0.02]  CS10Rot=[0 0 0]  CS11Pos=[]  CS11Rot=[]  CS12Pos=[]  CS12Rot=[]  CS13Pos=[]  CS13Rot=[]  CS14Pos=[]  CS14Rot=[]  CS15Pos=[]  CS15Rot=[]  CS16Pos=[]  CS16Rot=[]  CS17Pos=[]  CS17Rot=[]  CS18Pos=[]  CS18Rot=[]  CS19Pos=[]  CS19Rot=[]  CS20Pos=[]  CS20Rot=[]
      settings: SourceProductName=Simscape Multibody  SourceProductBaseCode=MS
  Demux : Demux  Outputs=6
  EndEffect Sensor_U : mblibv1/Sensors &  Actuators/Body Sensor  UpdateFromCAD=off  PhysicalDomain=Mechanical  PortType=blob  Muxed=on  Pose=off  Angle=on  AngleUnits=deg  ArcVelocity=on  ArcVelocityUnits=rad/s  ArcAcceleration=off  ArcAccelerationUnits=deg/s^2  CoordPosition=off  CoordPositionUnits=m  Velocity=on  VelocityUnits=m/s  Acceleration=off  AccelerationUnits=m/s^2  Quaternion=on  QuaternionDT=off  QuaternionDDT=off  QuaternionUnits=off  OutputVector=[1]  ActiveIO=on  Width=6  DialogClass=MechanicalSensorBlock  ReferenceFrame=Absolute (World)
      settings: SourceProductName=Simscape Multibody  SourceProductBaseCode=MS
  Force : MATLAB Function  TreatAsAtomicUnit=on
  Ground : mblibv1/Bodies/Ground  UpdateFromCAD=off  LeftPortType=env  RightPortType=workingframe  PhysicalDomain=Mechanical  DialogClass=GroundBlock  CoordPosition=[0 0 0]  CoordPositionUnits=m  StateVectorMgrId=0  MachineId=[1 0]  ShowEnvPort=on  ParameterChecksum=[284013180, 2921924473, 1228499562, 2456776883]  TopologyChecksum=[614394678, 2096192276, 1043109811, 1865987030]
      settings: SourceProductName=Simscape Multibody  SourceProductBaseCode=MS
  It : Constant  Value=120
  Joint Actuator_D1 : mblibv1/Sensors &  Actuators/Joint Actuator  UpdateFromCAD=off  PhysicalDomain=Mechanical  PortType=blob  ActuationStyle=Force  AngleUnits=deg  ArcVelocityUnits=deg/s  ArcAccelerationUnits=deg/s^2  CoordPositionUnits=m  VelocityUnits=m/s  AccelerationUnits=m/s^2  ForceUnits=N  TorqueUnits=N-m  ActiveIO=on  Width=1  DialogClass=MechanicalActuatorBlock  Primitive=R1  ReferenceFrame=Absolute (World)
      settings: SourceProductName=Simscape Multibody  SourceProductBaseCode=MS
  Joint Actuator_D2 : mblibv1/Sensors &  Actuators/Joint Actuator  UpdateFromCAD=off  PhysicalDomain=Mechanical  PortType=blob  ActuationStyle=Force  AngleUnits=deg  ArcVelocityUnits=deg/s  ArcAccelerationUnits=deg/s^2  CoordPositionUnits=m  VelocityUnits=m/s  AccelerationUnits=m/s^2  ForceUnits=N  TorqueUnits=N-m  ActiveIO=on  Width=1  DialogClass=MechanicalActuatorBlock  Primitive=R1  ReferenceFrame=Absolute (World)
      settings: SourceProductName=Simscape Multibody  SourceProductBaseCode=MS
  Joint Actuator_D3 : mblibv1/Sensors &  Actuators/Joint Actuator  UpdateFromCAD=off  PhysicalDomain=Mechanical  PortType=blob  ActuationStyle=Force  AngleUnits=deg  ArcVelocityUnits=deg/s  ArcAccelerationUnits=deg/s^2  CoordPositionUnits=m  VelocityUnits=m/s  AccelerationUnits=m/s^2  ForceUnits=N  TorqueUnits=N-m  ActiveIO=on  Width=1  DialogClass=MechanicalActuatorBlock  Primitive=R1  ReferenceFrame=Absolute (World)
      settings: SourceProductName=Simscape Multibody  SourceProductBaseCode=MS
  Joint Actuator_U1 : mblibv1/Sensors &  Actuators/Joint Actuator  UpdateFromCAD=off  PhysicalDomain=Mechanical  PortType=blob  ActuationStyle=Force  AngleUnits=deg  ArcVelocityUnits=deg/s  ArcAccelerationUnits=deg/s^2  CoordPositionUnits=m  VelocityUnits=m/s  AccelerationUnits=m/s^2  ForceUnits=N  TorqueUnits=N-m  ActiveIO=on  Width=1  DialogClass=MechanicalActuatorBlock  Primitive=R1  ReferenceFrame=Absolute (World)
      settings: SourceProductName=Simscape Multibody  SourceProductBaseCode=MS
  Joint Actuator_U2 : mblibv1/Sensors &  Actuators/Joint Actuator  UpdateFromCAD=off  PhysicalDomain=Mechanical  PortType=blob  ActuationStyle=Force  AngleUnits=deg  ArcVelocityUnits=deg/s  ArcAccelerationUnits=deg/s^2  CoordPositionUnits=m  VelocityUnits=m/s  AccelerationUnits=m/s^2  ForceUnits=N  TorqueUnits=N-m  ActiveIO=on  Width=1  DialogClass=MechanicalActuatorBlock  Primitive=R1  ReferenceFrame=Absolute (World)
      settings: SourceProductName=Simscape Multibody  SourceProductBaseCode=MS
  Joint Actuator_U3 : mblibv1/Sensors &  Actuators/Joint Actuator  UpdateFromCAD=off  PhysicalDomain=Mechanical  PortType=blob  ActuationStyle=Force  AngleUnits=deg  ArcVelocityUnits=deg/s  ArcAccelerationUnits=deg/s^2  CoordPositionUnits=m  VelocityUnits=m/s  AccelerationUnits=m/s^2  ForceUnits=N  TorqueUnits=N-m  ActiveIO=on  Width=1  DialogClass=MechanicalActuatorBlock  Primitive=R1  ReferenceFrame=Absolute (World)
      settings: SourceProductName=Simscape Multibody  SourceProductBaseCode=MS
  Joint Sensor_D1 : mblibv1/Sensors &  Actuators/Joint Sensor  UpdateFromCAD=off  PhysicalDomain=Mechanical  PortType=blob  Muxed=off  Pose=off  Angle=on  AngleUnits=rad  ArcVelocity=on  ArcVelocityUnits=rad/s  ArcAcceleration=off  ArcAccelerationUnits=rad/s^2  CoordPosition=on  CoordPositionUnits=m  Velocity=off  VelocityUnits=m/s  Acceleration=off  AccelerationUnits=m/s^2  Quaternion=on  QuaternionDT=off  QuaternionDDT=off  QuaternionUnits=off  OutputVector=[1]  ActiveIO=on  Width=2  DialogClass=MechanicalSensorBlock  Primitive=R1  Force=off  ForceUnits=N  Torque=off  TorqueUnits=N*m  ReferenceFrame=Absolute (World)  ReactionSensedSide=Base  ReactionReferenceFrame=Absolute (World)  ReactionForce=off  ReactionForceUnits=N  ReactionMoment=off  ReactionMomentUnits=N*m
      settings: SourceProductName=Simscape Multibody  SourceProductBaseCode=MS
  Joint Sensor_L2 : mblibv1/Sensors &  Actuators/Joint Sensor  UpdateFromCAD=off  PhysicalDomain=Mechanical  PortType=blob  Muxed=off  Pose=off  Angle=on  AngleUnits=rad  ArcVelocity=on  ArcVelocityUnits=rad/s  ArcAcceleration=off  ArcAccelerationUnits=rad/s^2  CoordPosition=on  CoordPositionUnits=m  Velocity=off  VelocityUnits=m/s  Acceleration=off  AccelerationUnits=m/s^2  Quaternion=on  QuaternionDT=off  QuaternionDDT=off  QuaternionUnits=off  OutputVector=[1]  ActiveIO=on  Width=2  DialogClass=MechanicalSensorBlock  Primitive=R1  Force=off  ForceUnits=N  Torque=off  TorqueUnits=N*m  ReferenceFrame=Absolute (World)  ReactionSensedSide=Base  ReactionReferenceFrame=Absolute (World)  ReactionForce=off  ReactionForceUnits=N  ReactionMoment=off  ReactionMomentUnits=N*m
      settings: SourceProductName=Simscape Multibody  SourceProductBaseCode=MS
  Joint Sensor_L3 : mblibv1/Sensors &  Actuators/Joint Sensor  UpdateFromCAD=off  PhysicalDomain=Mechanical  PortType=blob  Muxed=off  Pose=off  Angle=on  AngleUnits=rad  ArcVelocity=on  ArcVelocityUnits=rad/s  ArcAcceleration=off  ArcAccelerationUnits=rad/s^2  CoordPosition=on  CoordPositionUnits=m  Velocity=off  VelocityUnits=m/s  Acceleration=off  AccelerationUnits=m/s^2  Quaternion=on  QuaternionDT=off  QuaternionDDT=off  QuaternionUnits=off  OutputVector=[1]  ActiveIO=on  Width=2  DialogClass=MechanicalSensorBlock  Primitive=R1  Force=off  ForceUnits=N  Torque=off  TorqueUnits=N*m  ReferenceFrame=Absolute (World)  ReactionSensedSide=Base  ReactionReferenceFrame=Absolute (World)  ReactionForce=off  ReactionForceUnits=N  ReactionMoment=off  ReactionMomentUnits=N*m
      settings: SourceProductName=Simscape Multibody  SourceProductBaseCode=MS
  Joint Sensor_R3 : mblibv1/Sensors &  Actuators/Joint Sensor  UpdateFromCAD=off  PhysicalDomain=Mechanical  PortType=blob  Muxed=off  Pose=off  Angle=on  AngleUnits=rad  ArcVelocity=on  ArcVelocityUnits=rad/s  ArcAcceleration=on  ArcAccelerationUnits=rad/s^2  CoordPosition=on  CoordPositionUnits=m  Velocity=off  VelocityUnits=m/s  Acceleration=off  AccelerationUnits=m/s^2  Quaternion=on  QuaternionDT=off  QuaternionDDT=off  QuaternionUnits=off  OutputVector=[1]  ActiveIO=on  Width=3  DialogClass=MechanicalSensorBlock  Primitive=R1  Force=off  ForceUnits=N  Torque=off  TorqueUnits=N*m  ReferenceFrame=Absolute (World)  ReactionSensedSide=Base  ReactionReferenceFrame=Absolute (World)  ReactionForce=off  ReactionForceUnits=N  ReactionMoment=off  ReactionMomentUnits=N*m
      settings: SourceProductName=Simscape Multibody  SourceProductBaseCode=MS
  Joint Sensor_U1 : mblibv1/Sensors &  Actuators/Joint Sensor  UpdateFromCAD=off  PhysicalDomain=Mechanical  PortType=blob  Muxed=off  Pose=off  Angle=on  AngleUnits=rad  ArcVelocity=on  ArcVelocityUnits=rad/s  ArcAcceleration=on  ArcAccelerationUnits=rad/s^2  CoordPosition=on  CoordPositionUnits=m  Velocity=off  VelocityUnits=m/s  Acceleration=off  AccelerationUnits=m/s^2  Quaternion=on  QuaternionDT=off  QuaternionDDT=off  QuaternionUnits=off  OutputVector=[1]  ActiveIO=on  Width=3  DialogClass=MechanicalSensorBlock  Primitive=R1  Force=off  ForceUnits=N  Torque=off  TorqueUnits=N*m  ReferenceFrame=Absolute (World)  ReactionSensedSide=Base  ReactionReferenceFrame=Absolute (World)  ReactionForce=off  ReactionForceUnits=N  ReactionMoment=off  ReactionMomentUnits=N*m
      settings: SourceProductName=Simscape Multibody  SourceProductBaseCode=MS
  Joint Sensor_U2 : mblibv1/Sensors &  Actuators/Joint Sensor  UpdateFromCAD=off  PhysicalDomain=Mechanical  PortType=blob  Muxed=off  Pose=off  Angle=on  AngleUnits=rad  ArcVelocity=on  ArcVelocityUnits=rad/s  ArcAcceleration=on  ArcAccelerationUnits=rad/s^2  CoordPosition=on  CoordPositionUnits=m  Velocity=off  VelocityUnits=m/s  Acceleration=off  AccelerationUnits=m/s^2  Quaternion=on  QuaternionDT=off  QuaternionDDT=off  QuaternionUnits=off  OutputVector=[1]  ActiveIO=on  Width=3  DialogClass=MechanicalSensorBlock  Primitive=R1  Force=off  ForceUnits=N  Torque=off  TorqueUnits=N*m  ReferenceFrame=Absolute (World)  ReactionSensedSide=Base  ReactionReferenceFrame=Absolute (World)  ReactionForce=off  ReactionForceUnits=N  ReactionMoment=off  ReactionMomentUnits=N*m
      settings: SourceProductName=Simscape Multibody  SourceProductBaseCode=MS
  Joint0 Initial : mblibv1/Sensors &  Actuators/Joint Initial Condition  UpdateFromCAD=off  LeftPortType=blob  RightPortType=blob  PhysicalDomain=mechanical  DialogClass=InitialConditionBlock  InitialConditions=P1$false$-0.0163$m$deg$0$m/s$deg/s#P2$false$-0.0575$m$deg$0$m/s$deg/s#P3$false$0$m$deg$0$m/s$deg/s#R1$true$-pi/9$m$rad$0$m/s$rad/s#R2$false$0$m$deg$0$m/s$deg/s#R3$false$0$m$deg$0$m/s$deg/s#S$false$0$m$deg$0$m/s$deg/s  P1PIC=0  P1VIC=0  P2PIC=0  P2VIC=0  P3PIC=0  P3VIC=0  R1PIC=-pi/9  R1VIC=0  R2PIC=0  R2VIC=0  R3PIC=0  R3VIC=0  SPIC=0  SVIC=0
      settings: SourceProductName=Simscape Multibody  SourceProductBaseCode=MS
  Joint0 Initial1 : mblibv1/Sensors &  Actuators/Joint Initial Condition  UpdateFromCAD=off  LeftPortType=blob  RightPortType=blob  PhysicalDomain=mechanical  DialogClass=InitialConditionBlock  InitialConditions=P1$false$-0.0163$m$deg$0$m/s$deg/s#P2$false$-0.0575$m$deg$0$m/s$deg/s#P3$false$0$m$deg$0$m/s$deg/s#R1$true$pi/4$m$rad$0$m/s$rad/s#R2$false$0$m$deg$0$m/s$deg/s#R3$false$0$m$deg$0$m/s$deg/s#S$false$0$m$deg$0$m/s$deg/s  P1PIC=0  P1VIC=0  P2PIC=0  P2VIC=0  P3PIC=0  P3VIC=0  R1PIC=pi/4  R1VIC=0  R2PIC=0  R2VIC=0  R3PIC=0  R3VIC=0  SPIC=0  SVIC=0
      settings: SourceProductName=Simscape Multibody  SourceProductBaseCode=MS
  Joint0 Initial2 : mblibv1/Sensors &  Actuators/Joint Initial Condition  UpdateFromCAD=off  LeftPortType=blob  RightPortType=blob  PhysicalDomain=mechanical  DialogClass=InitialConditionBlock  InitialConditions=P1$false$-0.0163$m$deg$0$m/s$deg/s#P2$false$-0.0575$m$deg$0$m/s$deg/s#P3$false$0$m$deg$0$m/s$deg/s#R1$true$-pi/3$m$rad$0$m/s$rad/s#R2$false$0$m$deg$0$m/s$deg/s#R3$false$0$m$deg$0$m/s$deg/s#S$false$0$m$deg$0$m/s$deg/s  P1PIC=0  P1VIC=0  P2PIC=0  P2VIC=0  P3PIC=0  P3VIC=0  R1PIC=-pi/3  R1VIC=0  R2PIC=0  R2VIC=0  R3PIC=0  R3VIC=0  SPIC=0  SVIC=0
      settings: SourceProductName=Simscape Multibody  SourceProductBaseCode=MS
  Joint0 Initial3 : mblibv1/Sensors &  Actuators/Joint Initial Condition  UpdateFromCAD=off  LeftPortType=blob  RightPortType=blob  PhysicalDomain=mechanical  DialogClass=InitialConditionBlock  InitialConditions=P1$false$-0.0163$m$deg$0$m/s$deg/s#P2$false$-0.0575$m$deg$0$m/s$deg/s#P3$false$0$m$deg$0$m/s$deg/s#R1$true$pi/4$m$rad$0$m/s$rad/s#R2$false$0$m$deg$0$m/s$deg/s#R3$false$0$m$deg$0$m/s$deg/s#S$false$0$m$deg$0$m/s$deg/s  P1PIC=0  P1VIC=0  P2PIC=0  P2VIC=0  P3PIC=0  P3VIC=0  R1PIC=pi/4  R1VIC=0  R2PIC=0  R2VIC=0  R3PIC=0  R3VIC=0  SPIC=0  SVIC=0
      settings: SourceProductName=Simscape Multibody  SourceProductBaseCode=MS
  Joint0 Initial4 : mblibv1/Sensors &  Actuators/Joint Initial Condition  UpdateFromCAD=off  LeftPortType=blob  RightPortType=blob  PhysicalDomain=mechanical  DialogClass=InitialConditionBlock  InitialConditions=P1$false$-0.0163$m$deg$0$m/s$deg/s#P2$false$-0.0575$m$deg$0$m/s$deg/s#P3$false$0$m$deg$0$m/s$deg/s#R1$true$-pi/18$m$rad$0.0$m/s$rad/s#R2$false$0$m$deg$0$m/s$deg/s#R3$false$0$m$deg$0$m/s$deg/s#S$false$0$m$deg$0$m/s$deg/s  P1PIC=0  P1VIC=0  P2PIC=0  P2VIC=0  P3PIC=0  P3VIC=0  R1PIC=-pi/18  R1VIC=0.0  R2PIC=0  R2VIC=0  R3PIC=0  R3VIC=0  SPIC=0  SVIC=0
      settings: SourceProductName=Simscape Multibody  SourceProductBaseCode=MS
  Joint0 Initial5 : mblibv1/Sensors &  Actuators/Joint Initial Condition  UpdateFromCAD=off  LeftPortType=blob  RightPortType=blob  PhysicalDomain=mechanical  DialogClass=InitialConditionBlock  InitialConditions=P1$false$-0.0163$m$deg$0$m/s$deg/s#P2$false$-0.0575$m$deg$0$m/s$deg/s#P3$false$0$m$deg$0$m/s$deg/s#R1$true$-pi/9$m$rad$0$m/s$rad/s#R2$false$0$m$deg$0$m/s$deg/s#R3$false$0$m$deg$0$m/s$deg/s#S$false$0$m$deg$0$m/s$deg/s  P1PIC=0  P1VIC=0  P2PIC=0  P2VIC=0  P3PIC=0  P3VIC=0  R1PIC=-pi/9  R1VIC=0  R2PIC=0  R2VIC=0  R3PIC=0  R3VIC=0  SPIC=0  SVIC=0
      settings: SourceProductName=Simscape Multibody  SourceProductBaseCode=MS
  Joint0 Initial6 : mblibv1/Sensors &  Actuators/Joint Initial Condition  UpdateFromCAD=off  LeftPortType=blob  RightPortType=blob  PhysicalDomain=mechanical  DialogClass=InitialConditionBlock  InitialConditions=P1$false$0$m$deg$0$m/s$deg/s#P2$false$0$m$deg$0$m/s$deg/s#P3$false$0$m$deg$0$m/s$deg/s#R1$true$0$m$rad$0$m/s$rad/s#R2$false$0$m$deg$0$m/s$deg/s#R3$false$0$m$deg$0$m/s$deg/s#S$false$0$m$deg$0$m/s$deg/s  P1PIC=0  P1VIC=0  P2PIC=0  P2VIC=0  P3PIC=0  P3VIC=0  R1PIC=0  R1VIC=0  R2PIC=0  R2VIC=0  R3PIC=0  R3VIC=0  SPIC=0  SVIC=0
      settings: SourceProductName=Simscape Multibody  SourceProductBaseCode=MS
  Machine Environment : mblibv1/Bodies/Machine Environment  PortType=env  PhysicalDomain=Mechanical  DialogTemplateClass=MECH.MachineEnvironment  SyncWhenCopied=off  Gravity=[0 0 0]  GravityUnits=m/s^2  GravityAsSignal=off  Dimensionality=Auto-detect  AnalysisType=Forward dynamics  LinearAssemblyTolerance=1e-3  LinearAssemblyToleranceUnits=m  AngularAssemblyTolerance=1e-3  AngularAssemblyToleranceUnits=rad  ConstraintSolverType=Stabilizing  ConstraintRelTolerance=1e-4  ConstraintAbsTolerance=1e-4  UseRobustSingularityHandling=off  RedundancyAnalysisToleranceType=Automatically select tolerance  RedundancyAnalysisTolerance=1e-14  StatePerturbationType=Fixed  PerturbationSize=1e-5  VisualizeMachine=on  BodyVisualizationType=Use model default body geometries  BodyColorSelMode=Use model default  DefaultBodyColor=[1 0 0]
      settings: SourceProductName=Simscape Multibody  SourceProductBaseCode=MS
  Omega : Constant  Value=0
  Ref : mblibv1/Bodies/Body  LConnTagsString=CG|CS1|CS13|CS12  RConnTagsString=CS3  UpdateFromCAD=off  DialogClass=MechanicalBodyBlock  Mass=120  MassUnits=kg  InertiaUnits=kg*m^2  Inertia=120.0*eye(3)  Shape=Cylinder  ShapeDims=[1 1]  ShapeUnits=m  ShapeUse=false  Density=1  DensityUnits=kg/m^3  DensityUse=false  GraphicsMode=MACHINE_DEFAULT  BodyColorSelMode=COLORPALETTE  BodyColor=[0.87059 0.4902 0]  AttachedToCS=CG  CG=Left$CG$[0.3 0 0]$CS1$CS1$m$[0 0 0]$Euler X-Y-Z$deg$WORLD$true$none  WorkingFrames=Left$CS1$[0 0.0 0]$Adjoining$Adjoining$m$[0 0 0]$Euler X-Y-Z$deg$WORLD$true$none#Left$CS13$[0.3 0.0 0.3]$CS1$CS1$m$[0 0 0]$Euler X-Y-Z$deg$WORLD$true$none#Left$CS12$[0.3 0.0 -0.3]$CS1$CS1$m$[0 0 0]$Euler X-Y-Z$deg$WORLD$true$none#Right$CS3$[0.3 0.0 0]$CS1$CS1$m$[0 0 0]$Euler X-Y-Z$deg$WORLD$true$none#Right$CS2$[0 -0.3 0]$CS1$CS1$m$[0 0 0]$Euler X-Y-Z$deg$WORLD$false$none#Right$CS11$[0.0 0.3 0.3]$CS1$CS1$m$[0 0 0]$Euler X-Y-Z$deg$WORLD$false$none#Right$CS10$[0.6 0.3 0.3]$CS1$CS1$m$[0 0 0]$Euler X-Y-Z$deg$WORLD$false$none#Right$CS9$[0.6 -0.3 0.3]$CS1$CS1$m$[0 0 0]$Euler X-Y-Z$deg$WORLD$false$none#Right$CS8$[0.0 -0.3 0.3]$CS1$CS1$m$[0 0 0]$Euler X-Y-Z$deg$WORLD$false$none#Right$CS7$[0.0 0.3 -0.3]$CS1$CS1$m$[0 0 0]$Euler X-Y-Z$deg$WORLD$false$none#Right$CS6$[0.6 0.3 -0.3]$CS1$CS1$m$[0 0 0]$Euler X-Y-Z$deg$WORLD$false$none#Right$CS5$[0.6 -0.3 -0.3]$CS1$CS1$m$[0 0 0]$Euler X-Y-Z$deg$WORLD$false$none#Right$CS4$[0.0 -0.3 -0.3]$CS1$CS1$m$[0 0 0]$Euler X-Y-Z$deg$WORLD$false$none  CGPos=[0.3 0 0]  CGRot=[0 0 0]  CS0Pos=[]  CS0Rot=[]  CS1Pos=[0 0.0 0]  CS1Rot=[0 0 0]  CS2Pos=[0 -0.3 0]  CS2Rot=[0 0 0]  CS3Pos=[0.3 0.0 0]  CS3Rot=[0 0 0]  CS4Pos=[0.0 -0.3 -0.3]  CS4Rot=[0 0 0]  CS5Pos=[0.6 -0.3 -0.3]  CS5Rot=[0 0 0]  CS6Pos=[0.6 0.3 -0.3]  CS6Rot=[0 0 0]  CS7Pos=[0.0 0.3 -0.3]  CS7Rot=[0 0 0]  CS8Pos=[0.0 -0.3 0.3]  CS8Rot=[0 0 0]  CS9Pos=[0.6 -0.3 0.3]  CS9Rot=[0 0 0]  CS10Pos=[0.6 0.3 0.3]  CS10Rot=[0 0 0]  CS11Pos=[0.0 0.3 0.3]  CS11Rot=[0 0 0]  CS12Pos=[0.3 0.0 -0.3]  CS12Rot=[0 0 0]  CS13Pos=[0.3 0.0 0.3]  CS13Rot=[0 0 0]  CS14Pos=[]  CS14Rot=[]  CS15Pos=[]  CS15Rot=[]  CS16Pos=[]  CS16Rot=[]  CS17Pos=[]  CS17Rot=[]  CS18Pos=[]  CS18Rot=[]  CS19Pos=[]  CS19Rot=[]  CS20Pos=[]  CS20Rot=[]
      settings: SourceProductName=Simscape Multibody  SourceProductBaseCode=MS
  Scope : Scope  NumInputPorts=6
  U_Joint1 : mblibv1/Joints/Revolute  LConnTagsString=__newl0|SA1|SA2  RConnTagsString=__newr0|SA1  UpdateFromCAD=off  NumSAPorts=3  CutJoint=off  MarkAsCut=off  Primitives=prismatic  PrimitiveProps=R1$World$[0 0 1]$revolute  DialogClass=JointBlock  R1Axis=[0 0 1]
      settings: SourceProductName=Simscape Multibody  SourceProductBaseCode=MS
  U_Joint2 : mblibv1/Joints/Revolute  LConnTagsString=__newl0|SA1|SA2  RConnTagsString=__newr0|SA1  UpdateFromCAD=off  NumSAPorts=3  CutJoint=off  MarkAsCut=off  Primitives=prismatic  PrimitiveProps=R1$World$[0 0 1]$revolute  DialogClass=JointBlock  R1Axis=[0 0 1]
      settings: SourceProductName=Simscape Multibody  SourceProductBaseCode=MS
  U_Joint3 : mblibv1/Joints/Revolute  LConnTagsString=__newl0|SA1|SA2  RConnTagsString=__newr0|SA1  UpdateFromCAD=off  NumSAPorts=3  CutJoint=off  MarkAsCut=off  Primitives=prismatic  PrimitiveProps=R1$World$[0 0 1]$revolute  DialogClass=JointBlock  R1Axis=[0 0 1]
      settings: SourceProductName=Simscape Multibody  SourceProductBaseCode=MS
  U_Link1 : mblibv1/Bodies/Body  LConnTagsString=CS2  RConnTagsString=CS1  UpdateFromCAD=off  DialogClass=MechanicalBodyBlock  Mass=2.49  MassUnits=kg  InertiaUnits=kg*m^2  Inertia=[0.208 0 0; 0 0.208 0;0 0 0.208]  Shape=Cylinder  ShapeDims=[1 1]  ShapeUnits=m  ShapeUse=false  Density=1  DensityUnits=kg/m^3  DensityUse=false  GraphicsMode=MACHINE_DEFAULT  BodyColorSelMode=COLORPALETTE  BodyColor=[0 0.6 0.6]  AttachedToCS=CG  CG=Right$CG$[0.2 0.0 0]$CS1$CS1$m$[0 0 0]$Euler X-Y-Z$deg$WORLD$false$none  WorkingFrames=Right$CS1$[0 0 0]$Adjoining$Adjoining$m$[0 0 0]$Euler X-Y-Z$deg$WORLD$true$none#Left$CS2$[0.4 0.0 0]$CS1$CS1$m$[0 0 0]$Euler X-Y-Z$deg$WORLD$true$none#Left$CS3$[0.4 0.02 0.02]$CS1$CS1$m$[0 0 0]$Euler X-Y-Z$deg$WORLD$false$none#Left$CS7$[0.0 0.02 0.02]$CS1$CS1$m$[0 0 0]$Euler X-Y-Z$deg$WORLD$false$none#Left$CS6$[0.4 -0.02 -0.02]$CS1$CS1$m$[0 0 0]$Euler X-Y-Z$deg$WORLD$false$none#Left$CS8$[0.0 -0.02 -0.02]$CS1$CS1$m$[0 0 0]$Euler X-Y-Z$deg$WORLD$false$none#Left$CS5$[0.4 0.02 -0.02]$CS1$CS1$m$[0 0 0]$Euler X-Y-Z$deg$WORLD$false$none#Left$CS9$[0.0 0.02 -0.02]$CS1$CS1$m$[0 0 0]$Euler X-Y-Z$deg$WORLD$false$none#Left$CS4$[0.4 -0.02 0.02]$CS1$CS1$m$[0 0 0]$Euler X-Y-Z$deg$WORLD$false$none#Left$CS10$[0.0 -0.02 0.02]$CS1$CS1$m$[0 0 0]$Euler X-Y-Z$deg$WORLD$false$none  CGPos=[0.2 0.0 0]  CGRot=[0 0 0]  CS0Pos=[]  CS0Rot=[]  CS1Pos=[0 0 0]  CS1Rot=[0 0 0]  CS2Pos=[0.4 0.0 0]  CS2Rot=[0 0 0]  CS3Pos=[0.4 0.02 0.02]  CS3Rot=[0 0 0]  CS4Pos=[0.4 -0.02 0.02]  CS4Rot=[0 0 0]  CS5Pos=[0.4 0.02 -0.02]  CS5Rot=[0 0 0]  CS6Pos=[0.4 -0.02 -0.02]  CS6Rot=[0 0 0]  CS7Pos=[0.0 0.02 0.02]  CS7Rot=[0 0 0]  CS8Pos=[0.0 -0.02 -0.02]  CS8Rot=[0 0 0]  CS9Pos=[0.0 0.02 -0.02]  CS9Rot=[0 0 0]  CS10Pos=[0.0 -0.02 0.02]  CS10Rot=[0 0 0]  CS11Pos=[]  CS11Rot=[]  CS12Pos=[]  CS12Rot=[]  CS13Pos=[]  CS13Rot=[]  CS14Pos=[]  CS14Rot=[]  CS15Pos=[]  CS15Rot=[]  CS16Pos=[]  CS16Rot=[]  CS17Pos=[]  CS17Rot=[]  CS18Pos=[]  CS18Rot=[]  CS19Pos=[]  CS19Rot=[]  CS20Pos=[]  CS20Rot=[]
      settings: SourceProductName=Simscape Multibody  SourceProductBaseCode=MS
  U_Link2 : mblibv1/Bodies/Body  LConnTagsString=CS2  RConnTagsString=CS1  UpdateFromCAD=off  DialogClass=MechanicalBodyBlock  Mass=2.49  MassUnits=kg  InertiaUnits=kg*m^2  Inertia=[0.208 0 0; 0 0.208 0;0 0 0.208]  Shape=Cylinder  ShapeDims=[1 1]  ShapeUnits=m  ShapeUse=false  Density=1  DensityUnits=kg/m^3  DensityUse=false  GraphicsMode=MACHINE_DEFAULT  BodyColorSelMode=COLORPALETTE  BodyColor=[0 1 0]  AttachedToCS=CG  CG=Right$CG$[0.2 0.0 0]$CS1$CS1$m$[0 0 0]$Euler X-Y-Z$deg$WORLD$false$none  WorkingFrames=Right$CS1$[0 0 0]$Adjoining$Adjoining$m$[0 0 0]$Euler X-Y-Z$deg$WORLD$true$none#Left$CS2$[0.4 0.0 0]$CS1$CS1$m$[0 0 0]$Euler X-Y-Z$deg$WORLD$true$none#Left$CS3$[0.4 0.02 0.02]$CS1$CS1$m$[0 0 0]$Euler X-Y-Z$deg$WORLD$false$none#Left$CS7$[0.0 0.02 0.02]$CS1$CS1$m$[0 0 0]$Euler X-Y-Z$deg$WORLD$false$none#Left$CS6$[0.4 -0.02 -0.02]$CS1$CS1$m$[0 0 0]$Euler X-Y-Z$deg$WORLD$false$none#Left$CS8$[0.0 -0.02 -0.02]$CS1$CS1$m$[0 0 0]$Euler X-Y-Z$deg$WORLD$false$none#Left$CS5$[0.4 0.02 -0.02]$CS1$CS1$m$[0 0 0]$Euler X-Y-Z$deg$WORLD$false$none#Left$CS9$[0.0 0.02 -0.02]$CS1$CS1$m$[0 0 0]$Euler X-Y-Z$deg$WORLD$false$none#Left$CS4$[0.4 -0.02 0.02]$CS1$CS1$m$[0 0 0]$Euler X-Y-Z$deg$WORLD$false$none#Left$CS10$[0.0 -0.02 0.02]$CS1$CS1$m$[0 0 0]$Euler X-Y-Z$deg$WORLD$false$none  CGPos=[0.2 0.0 0]  CGRot=[0 0 0]  CS0Pos=[]  CS0Rot=[]  CS1Pos=[0 0 0]  CS1Rot=[0 0 0]  CS2Pos=[0.4 0.0 0]  CS2Rot=[0 0 0]  CS3Pos=[0.4 0.02 0.02]  CS3Rot=[0 0 0]  CS4Pos=[0.4 -0.02 0.02]  CS4Rot=[0 0 0]  CS5Pos=[0.4 0.02 -0.02]  CS5Rot=[0 0 0]  CS6Pos=[0.4 -0.02 -0.02]  CS6Rot=[0 0 0]  CS7Pos=[0.0 0.02 0.02]  CS7Rot=[0 0 0]  CS8Pos=[0.0 -0.02 -0.02]  CS8Rot=[0 0 0]  CS9Pos=[0.0 0.02 -0.02]  CS9Rot=[0 0 0]  CS10Pos=[0.0 -0.02 0.02]  CS10Rot=[0 0 0]  CS11Pos=[]  CS11Rot=[]  CS12Pos=[]  CS12Rot=[]  CS13Pos=[]  CS13Rot=[]  CS14Pos=[]  CS14Rot=[]  CS15Pos=[]  CS15Rot=[]  CS16Pos=[]  CS16Rot=[]  CS17Pos=[]  CS17Rot=[]  CS18Pos=[]  CS18Rot=[]  CS19Pos=[]  CS19Rot=[]  CS20Pos=[]  CS20Rot=[]
      settings: SourceProductName=Simscape Multibody  SourceProductBaseCode=MS
  U_Link3 : mblibv1/Bodies/Body  LConnTagsString=CS2|CS3  RConnTagsString=CG|CS1  UpdateFromCAD=off  DialogClass=MechanicalBodyBlock  Mass=2.49  MassUnits=kg  InertiaUnits=kg*m^2  Inertia=[0.208 0 0; 0 0.208 0;0 0 0.208]  Shape=Cylinder  ShapeDims=[1 1]  ShapeUnits=m  ShapeUse=false  Density=1  DensityUnits=kg/m^3  DensityUse=false  GraphicsMode=MACHINE_DEFAULT  BodyColorSelMode=MACHINE_DEFAULT  BodyColor=[1 0 0]  AttachedToCS=CG  CG=Right$CG$[0.2 0.0 0]$CS1$CS1$m$[0 0 0]$Euler X-Y-Z$deg$WORLD$true$none  WorkingFrames=Right$CS1$[0 0 0]$Adjoining$Adjoining$m$[0 0 0]$Euler X-Y-Z$deg$WORLD$true$none#Left$CS2$[0.4 0.0 0]$CS1$CS1$m$[0 0 0]$Euler X-Y-Z$deg$WORLD$true$none#Left$CS3$[0.4 0.0 0]$CS1$CS1$m$[0 0 0]$Euler X-Y-Z$deg$WORLD$true$none#Left$CS4$[0.4 0.02 0.02]$CS1$CS1$m$[0 0 0]$Euler X-Y-Z$deg$WORLD$false$none#Left$CS7$[0.4 0.02 -0.02]$CS1$CS1$m$[0 0 0]$Euler X-Y-Z$deg$WORLD$false$none#Left$CS6$[0.4 -0.02 0.02]$CS1$CS1$m$[0 0 0]$Euler X-Y-Z$deg$WORLD$false$none#Left$CS5$[0.4 -0.02 -0.02]$CS1$CS1$m$[0 0 0]$Euler X-Y-Z$deg$WORLD$false$none#Left$CS11$[0.0 -0.02 0.02]$CS1$CS1$m$[0 0 0]$Euler X-Y-Z$deg$WORLD$false$none#Left$CS10$[0.0 -0.02 -0.02]$CS1$CS1$m$[0 0 0]$Euler X-Y-Z$deg$WORLD$false$none#Left$CS9$[0.0 0.02 -0.02]$CS1$CS1$m$[0 0 0]$Euler X-Y-Z$deg$WORLD$false$none#Left$CS8$[0.0 0.02 0.02]$CS1$CS1$m$[0 0 0]$Euler X-Y-Z$deg$WORLD$false$none  CGPos=[0.2 0.0 0]  CGRot=[0 0 0]  CS0Pos=[]  CS0Rot=[]  CS1Pos=[0 0 0]  CS1Rot=[0 0 0]  CS2Pos=[0.4 0.0 0]  CS2Rot=[0 0 0]  CS3Pos=[0.4 0.0 0]  CS3Rot=[0 0 0]  CS4Pos=[0.4 0.02 0.02]  CS4Rot=[0 0 0]  CS5Pos=[0.4 -0.02 -0.02]  CS5Rot=[0 0 0]  CS6Pos=[0.4 -0.02 0.02]  CS6Rot=[0 0 0]  CS7Pos=[0.4 0.02 -0.02]  CS7Rot=[0 0 0]  CS8Pos=[0.0 0.02 0.02]  CS8Rot=[0 0 0]  CS9Pos=[0.0 0.02 -0.02]  CS9Rot=[0 0 0]  CS10Pos=[0.0 -0.02 -0.02]  CS10Rot=[0 0 0]  CS11Pos=[0.0 -0.02 0.02]  CS11Rot=[0 0 0]  CS12Pos=[]  CS12Rot=[]  CS13Pos=[]  CS13Rot=[]  CS14Pos=[]  CS14Rot=[]  CS15Pos=[]  CS15Rot=[]  CS16Pos=[]  CS16Rot=[]  CS17Pos=[]  CS17Rot=[]  CS18Pos=[]  CS18Rot=[]  CS19Pos=[]  CS19Rot=[]  CS20Pos=[]  CS20Rot=[]
      settings: SourceProductName=Simscape Multibody  SourceProductBaseCode=MS
  Weld{,1..8} (9 alike) : mblibv1/Joints/Weld  LConnTagsString=__newl0  RConnTagsString=__newr0  UpdateFromCAD=off  NumSAPorts=0  CutJoint=off  MarkAsCut=off  Primitives=weld  PrimitiveProps=W$WORLD$[0 0 0]$weld  DialogClass=JointBlock  WAxis=[0 0 0]
      settings: SourceProductName=Simscape Multibody  SourceProductBaseCode=MS
  r_3U : Scope
  Link_Ang_D1 : Outport
  Link_Ang_D2 : Outport  Port=2
  Link_Ang_D3 : Outport  Port=3
  Link_Ang_D1_w : Outport  Port=4
  Link_Ang_D2_w : Outport  Port=5
  Link_Ang_D3_w : Outport  Port=6
  Base_Ang : Outport  Port=7
  Base_Ang_w : Outport  Port=8
  Link_Ang_U1 : Outport  Port=9
  EndEffect_U_ve_w : Outport  Port=10
  Link_Ang_U2 : Outport  Port=11
  Link_Ang_U3 : Outport  Port=12
  Link_Ang_U1_w : Outport  Port=13
  Link_Ang_U2_w : Outport  Port=14
  Link_Ang_U3_w : Outport  Port=15
  r_0 : Outport  Port=16
  Target_p_v_w : Outport  Port=17
  Link_Ang_U1_a : Outport  Port=18
  Link_Ang_U2_a : Outport  Port=19
  Link_Ang_U3_a : Outport  Port=20
  wires:
  Joint Sensor_D1/1 -> Link_Ang_D1/1
  Link_Actuator_D1/1 -> Joint Actuator_D1/1
  Joint Sensor_L2/1 -> Link_Ang_D2/1
  Joint Sensor_L3/1 -> Link_Ang_D3/1
  Link_Actuator_D2/1 -> Joint Actuator_D2/1
  Link_Actuator_D3/1 -> Joint Actuator_D3/1
  Joint Sensor_D1/2 -> Link_Ang_D1_w/1
  Joint Sensor_L2/2 -> Link_Ang_D2_w/1
  Joint Sensor_L3/2 -> Link_Ang_D3_w/1
  Base Sensor_x/1 -> Base_x_p/1
  Base Sensor_y/1 -> Base_y_p/1
  Base Sensor_ang_Tc/1 -> Base_Ang/1
  Base Sensor_x/2 -> Base_x_v/1
  Base Sensor_y/2 -> Base_y_v/1
  Base Sensor_ang_Tc/2 -> Base_Ang_w/1
  Joint Sensor_U1/1 -> Link_Ang_U1/1
  EndEffect Sensor_U/1 -> EndEffect_U_ve_w/1
  Link_Actuator_U1/1 -> Joint Actuator_U1/1
  Joint Sensor_U2/1 -> Link_Ang_U2/1
  Joint Sensor_R3/1 -> Link_Ang_U3/1
  Link_Actuator_U2/1 -> Joint Actuator_U2/1
  Link_Actuator_U3/1 -> Joint Actuator_U3/1
  Joint Sensor_U1/2 -> Link_Ang_U1_w/1
  Joint Sensor_U2/2 -> Link_Ang_U2_w/1
  Joint Sensor_R3/2 -> Link_Ang_U3_w/1
  Body Sensor/1 -> r_0/1
  Body Sensor5/1 -> r_3U/1
  Body Sensor2/1 -> Target_p_v_w/1
  Force/1(F) -> Demux/1, Body Actuator/1
  Counter/1 -> Force/1(counter)
  Demux/1 -> Scope/1
  Demux/2 -> Scope/2
  Demux/6 -> Scope/6
  Demux/5 -> Scope/5
  Demux/4 -> Scope/4
  Demux/3 -> Scope/3
  Omega/1 -> Force/2(omega)
  It/1 -> Force/3(It)
  Joint Sensor_U1/3 -> Link_Ang_U1_a/1
  Joint Sensor_U2/3 -> Link_Ang_U2_a/1
  Joint Sensor_R3/3 -> Link_Ang_U3_a/1
  connections:
  Custom Joint/RConn1 -- Base/LConn4
  D_Joint1/LConn1 -- Base/RConn2
  U_Joint1/LConn1 -- Base/RConn1
  Ground/RConn1 -- Custom Joint/LConn1
  EndEffect Sensor_U/LConn1 -- U_Link3/LConn1
  Machine Environment/RConn1 -- Ground/LConn1
  Joint Actuator_D1/RConn1 -- D_Joint1/LConn2
  Joint Actuator_D2/RConn1 -- D_Joint2/LConn2
  Joint Actuator_D3/RConn1 -- D_Joint3/LConn2
  Joint Actuator_U1/RConn1 -- U_Joint1/LConn2
  Joint Actuator_U2/RConn1 -- U_Joint2/LConn2
  Joint Actuator_U3/RConn1 -- U_Joint3/LConn2
  Joint Sensor_D1/LConn1 -- D_Joint1/RConn2
  Joint Sensor_L2/LConn1 -- D_Joint2/RConn2
  Joint Sensor_L3/LConn1 -- D_Joint3/RConn2
  Joint Sensor_U2/LConn1 -- U_Joint2/RConn2
  Joint Sensor_R3/LConn1 -- U_Joint3/RConn2
  D_Link1/RConn1 -- D_Joint1/RConn1
  D_Joint2/LConn1 -- D_Link1/LConn1
  D_Link2/RConn1 -- D_Joint2/RConn1
  D_Joint3/LConn1 -- D_Link2/LConn1
  D_Joint3/RConn1 -- D_Link3/RConn1
  U_Joint1/RConn1 -- U_Link1/RConn1
  U_Link1/LConn1 -- U_Joint2/LConn1
  U_Link2/RConn1 -- U_Joint2/RConn1
  U_Joint3/LConn1 -- U_Link2/LConn1
  U_Joint3/RConn1 -- U_Link3/RConn2
  Base Sensor_y/LConn1 -- Custom Joint/LConn3
  Custom Joint/RConn2 -- Base Sensor_ang_Tc/LConn1
  U_Joint1/RConn2 -- Joint Sensor_U1/LConn1
  Joint0 Initial/RConn1 -- D_Joint1/LConn3
  Joint0 Initial1/RConn1 -- D_Joint2/LConn3
  Joint0 Initial2/RConn1 -- D_Joint3/LConn3
  Joint0 Initial3/RConn1 -- U_Joint1/LConn3
  Joint0 Initial5/RConn1 -- U_Joint3/LConn3
  Joint0 Initial4/RConn1 -- U_Joint2/LConn3
  Joint0 Initial6/RConn1 -- Custom Joint/RConn3
  Base/LConn2 -- Weld/LConn1
  Base/LConn3 -- Weld1/LConn1
  Weld/RConn1 -- Body/LConn1
  Weld2/LConn1 -- Body/RConn1
  Weld2/RConn1 -- Body1/LConn1
  Body3/LConn1 -- Weld3/RConn1
  Weld1/RConn1 -- Body2/LConn1
  Weld3/LConn1 -- Body2/RConn1
  Base/LConn1 -- Body Sensor/LConn1
  U_Link3/RConn1 -- Body Sensor5/LConn1
  Weld4/RConn1 -- Body4/LConn1
  Weld6/LConn1 -- Ref/LConn4
  Weld4/LConn1 -- Ref/LConn3
  Weld6/RConn1 -- Body6/LConn1
  Body7/LConn1 -- Weld7/RConn1
  Ref/RConn1 -- Body Sensor2/LConn1
  Weld7/LConn1 -- Body6/RConn1
  Weld5/RConn1 -- Body5/LConn1
  Weld5/LConn1 -- Body4/RConn1
  U_Link3/LConn2 -- Weld8/LConn1
  Weld8/RConn1 -- Ref/LConn2
  Body Actuator/RConn1 -- Ref/LConn1
  Base Sensor_x/LConn1 -- Custom Joint/LConn2
